simulink model "NDR"  (R2025b)
settings: Solver=VariableStepAuto  StartTime=0.0  StopTime=10.0  RelTol=1e-6
settings Model: Creator=arxchy  LastModifiedBy=arxchy

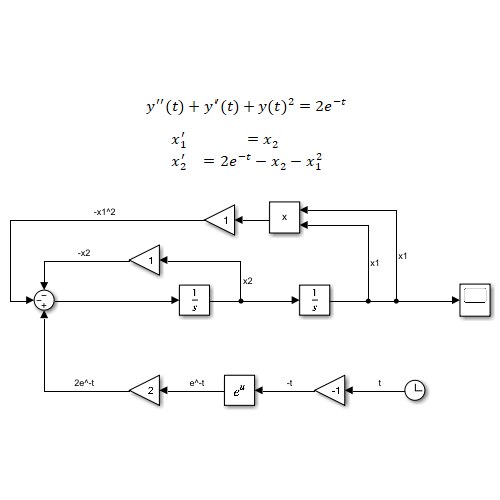
[thumbnail: Simulink's stored preview of the top-level diagram]
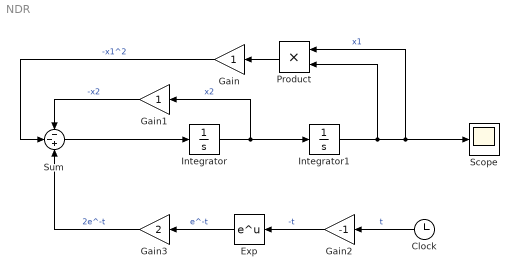
== system NDR ==
  Clock : Clock
  Exp : Math
  Gain : Gain
  Gain1 : Gain
  Gain2 : Gain  Gain=-1
  Gain3 : Gain  Gain=2
  Integrator : Integrator  InitialCondition=1
  Integrator1 : Integrator
  Product : Product
  Scope : Scope
      settings: ActiveDisplayYMinimum=-0.18914698105563721  ActiveDisplayYMaximum=1.4648788259606318
  Sum : Sum  Inputs=--+
  wires:
  Integrator/1 -> Gain1/1, Integrator1/1  "x2"
  Integrator1/1 -> Product/2, Product/1, Scope/1  "x1"
  Gain/1 -> Sum/2  "-x1^2"
  Gain1/1 -> Sum/1  "-x2"
  Sum/1 -> Integrator/1
  Exp/1 -> Gain3/1  "e^-t"
  Gain2/1 -> Exp/1  "-t"
  Clock/1 -> Gain2/1  "t"
  Gain3/1 -> Sum/3  "2e^-t"
  Product/1 -> Gain/1
